simulink model "ManobraOrbital"  (R2023b)
settings: Solver=FixedStepAuto  StartTime=0.0  StopTime=tf  FixedStep=step_modelo  RelTol=1e-3
values from neighbouring files (symbols this model uses):
  mi = 3.9860044189*10^14    (= 398600441890000)    [constantes.m]
undefined symbols (not defined in the file or in its folder): e0_ini, pcoRad, step_modelo, t_man, x0_dot, x0_dot_ini, x0_ini, y0_dot_ini, y0_ini, z0_dot_ini, z0_ini
libraries: simulink x5
settings Model: Creator=rodri  LastModifiedBy=rodri
settings DataIOCC: SaveOutput=off  SaveTime=off
settings ModelReferenceCC: EnableRefExpFcnMdlSchedulingChecks=on

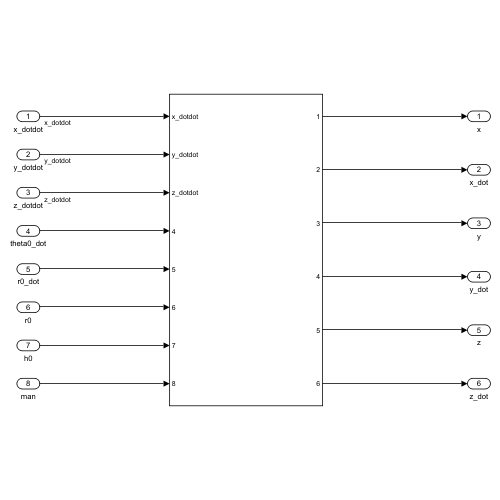
[thumbnail: Simulink's stored preview of the top-level diagram]
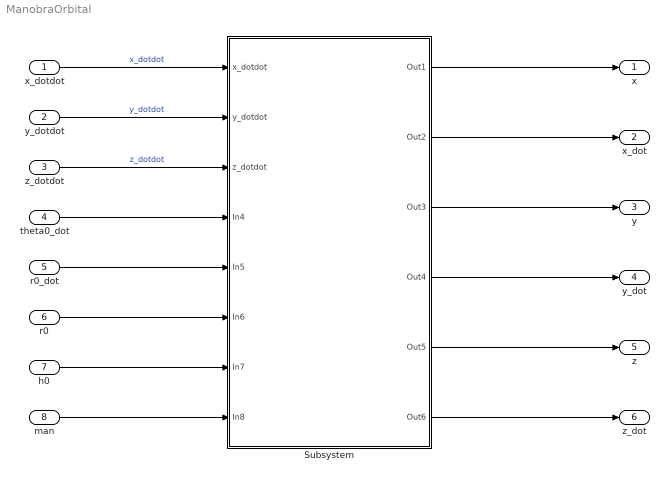
== system ManobraOrbital ==
  x_dotdot : Inport  OutDataTypeStr=double  Interpolate=off
  y_dotdot : Inport  Port=2  OutDataTypeStr=double  Interpolate=off
  z_dotdot : Inport  Port=3  OutDataTypeStr=double  Interpolate=off
  theta0_dot : Inport  Port=4  OutDataTypeStr=double  Interpolate=off
  r0_dot : Inport  Port=5  OutDataTypeStr=double  Interpolate=off
  r0 : Inport  Port=6  OutDataTypeStr=double  Interpolate=off
  h0 : Inport  Port=7  OutDataTypeStr=double  Interpolate=off
  man : Inport  Port=8  OutDataTypeStr=boolean
  Subsystem : Subsystem
  x : Outport  OutDataTypeStr=double
  x_dot : Outport  Port=2  OutDataTypeStr=double
  y : Outport  Port=3  OutDataTypeStr=double
  y_dot : Outport  Port=4  OutDataTypeStr=double
  z : Outport  Port=5  OutDataTypeStr=double
  z_dot : Outport  Port=6  OutDataTypeStr=double
  wires:
  x_dotdot/1 -> Subsystem/1(x_dotdot)  "x_dotdot"
  y_dotdot/1 -> Subsystem/2(y_dotdot)  "y_dotdot"
  z_dotdot/1 -> Subsystem/3(z_dotdot)  "z_dotdot"
  theta0_dot/1 -> Subsystem/4(In4)
  r0_dot/1 -> Subsystem/5(In5)
  r0/1 -> Subsystem/6(In6)
  h0/1 -> Subsystem/7(In7)
  man/1 -> Subsystem/8(In8)
  Subsystem/1(Out1) -> x/1
  Subsystem/2(Out2) -> x_dot/1
  Subsystem/3(Out3) -> y/1
  Subsystem/4(Out4) -> y_dot/1
  Subsystem/5(Out5) -> z/1
  Subsystem/6(Out6) -> z_dot/1

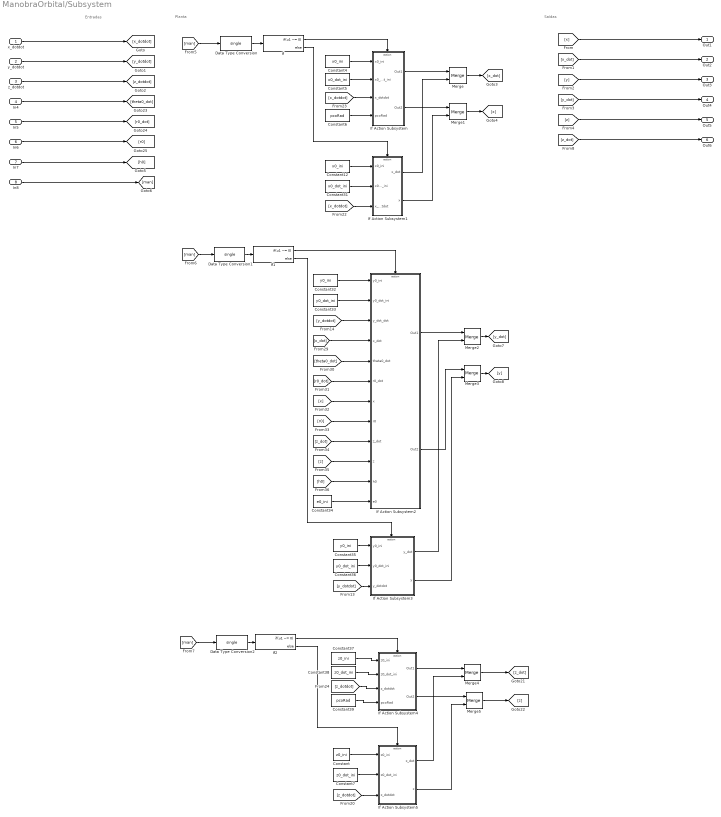
== system ManobraOrbital/Subsystem ==
  note: Planta
  note: Entradas
  note: Saídas
  x_dotdot : Inport
  y_dotdot : Inport  Port=2
  z_dotdot : Inport  Port=3
  In4 : Inport  Port=4
  In5 : Inport  Port=5
  In6 : Inport  Port=6
  In7 : Inport  Port=7
  In8 : Inport  Port=8
  Constant : Constant  Value=z0_ini  SampleTime=-1
  Constant12 : Constant  Value=x0_ini  SampleTime=-1
  Constant31 : Constant  Value=x0_dot_ini  SampleTime=-1
  Constant32 : Constant  Value=y0_ini  SampleTime=-1
  Constant33 : Constant  Value=y0_dot_ini  SampleTime=-1
  Constant34 : Constant  Value=e0_ini  SampleTime=-1  LockScale=on
  Constant35 : Constant  Value=y0_ini  SampleTime=-1
  Constant36 : Constant  Value=y0_dot_ini  SampleTime=-1
  Constant37 : Constant  Value=z0_ini  SampleTime=-1
  Constant38 : Constant  Value=z0_dot_ini  SampleTime=-1
  Constant39 : Constant  Value=pcoRad  SampleTime=-1
  Constant4 : Constant  Value=x0_ini  SampleTime=-1
  Constant5 : Constant  Value=x0_dot_ini  SampleTime=-1
  Constant6 : Constant  Value=pcoRad  SampleTime=-1
  Constant7 : Constant  Value=z0_dot_ini  SampleTime=-1
  Data Type Conversion : DataTypeConversion  OutDataTypeStr=single  SaturateOnIntegerOverflow=off  RndMeth=Floor
  Data Type Conversion1 : DataTypeConversion  OutDataTypeStr=single  SaturateOnIntegerOverflow=off  RndMeth=Floor
  Data Type Conversion2 : DataTypeConversion  OutDataTypeStr=single  SaturateOnIntegerOverflow=off  RndMeth=Floor
  If : If  IfExpression=u1 ~= 0
  If Action Subsystem : Subsystem  TreatAsAtomicUnit=on
  If Action Subsystem1 : Subsystem  TreatAsAtomicUnit=on
  If Action Subsystem2 : Subsystem  TreatAsAtomicUnit=on
  If Action Subsystem3 : Subsystem  TreatAsAtomicUnit=on
  If Action Subsystem4 : Subsystem  TreatAsAtomicUnit=on
  If Action Subsystem5 : Subsystem  TreatAsAtomicUnit=on
  If1 : If  IfExpression=u1 ~= 0
  If2 : If  IfExpression=u1 ~= 0
  Merge : Merge  InitialOutput=x0_dot_ini
  Merge1 : Merge  InitialOutput=x0_ini
  Merge2 : Merge  InitialOutput=y0_dot_ini
  Merge3 : Merge  InitialOutput=y0_ini
  Merge4 : Merge  InitialOutput=z0_dot_ini
  Merge5 : Merge  InitialOutput=z0_ini
  Out1 : Outport
  Out2 : Outport  Port=2
  Out3 : Outport  Port=3
  Out4 : Outport  Port=4
  Out5 : Outport  Port=5
  Out6 : Outport  Port=6
  wires:
  [y_dotdot] -> If Action Subsystem2/3(y_dot_dot)
  Merge/1 -> [x_dot]
  If Action Subsystem4/2(Out2) -> Merge5/1
  Constant5/1 -> If Action Subsystem/2(x0_dot_ini)
  Constant37/1 -> If Action Subsystem4/1(z0_ini)
  [x] -> Out1/1
  Constant7/1 -> If Action Subsystem5/2(z0_dot_ini)
  [r0] -> If Action Subsystem2/8(r0)
  If2/2 -> If Action Subsystem5/Action
  If Action Subsystem/2(Out2) -> Merge1/1
  [z_dotdot] -> If Action Subsystem5/3(z_dotdot)
  [z_dot] -> Out6/1
  Constant32/1 -> If Action Subsystem2/1(y0_ini)
  [h0] -> If Action Subsystem2/11(h0)
  In8/1 -> [man]
  If1/2 -> If Action Subsystem3/Action
  Constant35/1 -> If Action Subsystem3/1(y0_ini)
  If1/1 -> If Action Subsystem2/Action
  [y_dotdot] -> If Action Subsystem3/3(y_dotdot)
  Data Type Conversion2/1 -> If2/1
  If Action Subsystem3/1(y_dot) -> Merge2/2
  In7/1 -> [h0]
  In5/1 -> [r0_dot]
  Merge2/1 -> [y_dot]
  Constant/1 -> If Action Subsystem5/1(z0_ini)
  If2/1 -> If Action Subsystem4/Action
  [r0_dot] -> If Action Subsystem2/6(r0_dot)
  If Action Subsystem1/1(x_dot) -> Merge/2
  [z] -> If Action Subsystem2/10(z)
  Constant34/1 -> If Action Subsystem2/12(e0)
  [x_dot] -> If Action Subsystem2/4(x_dot)
  Constant36/1 -> If Action Subsystem3/2(y0_dot_ini)
  [theta0_dot] -> If Action Subsystem2/5(theta0_dot)
  Data Type Conversion1/1 -> If1/1
  Merge3/1 -> [y]
  [man] -> Data Type Conversion1/1
  Merge1/1 -> [x]
  If Action Subsystem2/1(Out1) -> Merge2/1
  If Action Subsystem4/1(Out1) -> Merge4/1
  Constant38/1 -> If Action Subsystem4/2(z0_dot_ini)
  Merge4/1 -> [z_dot]
  [x_dotdot] -> If Action Subsystem1/3(x_dotdot)
  If Action Subsystem/1(Out1) -> Merge/1
  [z_dotdot] -> If Action Subsystem4/3(z_dotdot)
  [z_dot] -> If Action Subsystem2/9(z_dot)
  If Action Subsystem2/2(Out2) -> Merge3/1
  If Action Subsystem1/2(x) -> Merge1/2
  Constant39/1 -> If Action Subsystem4/4(pcoRad)
  If Action Subsystem3/2(y) -> Merge3/2
  Constant31/1 -> If Action Subsystem1/2(x0_dot_ini)
  Constant4/1 -> If Action Subsystem/1(x0_ini)
  If/1 -> If Action Subsystem/Action
  [man] -> Data Type Conversion/1
  Data Type Conversion/1 -> If/1
  Constant12/1 -> If Action Subsystem1/1(x0_ini)
  Merge5/1 -> [z]
  Constant6/1 -> If Action Subsystem/4(pcoRad)
  If/2 -> If Action Subsystem1/Action
  [x_dot] -> Out2/1
  [x] -> If Action Subsystem2/7(x)
  Constant33/1 -> If Action Subsystem2/2(y0_dot_ini)
  [man] -> Data Type Conversion2/1
  If Action Subsystem5/1(z_dot) -> Merge4/2
  y_dotdot/1 -> [y_dotdot]
  If Action Subsystem5/2(z) -> Merge5/2
  [x_dotdot] -> If Action Subsystem/3(x_dotdot)
  In6/1 -> [r0]
  [z] -> Out5/1
  x_dotdot/1 -> [x_dotdot]
  z_dotdot/1 -> [z_dotdot]
  [y] -> Out3/1
  In4/1 -> [theta0_dot]
  [y_dot] -> Out4/1

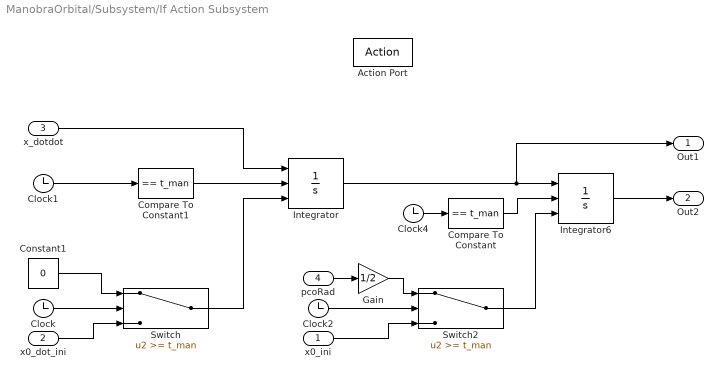
== system ManobraOrbital/Subsystem/If Action Subsystem ==
  x0_ini : Inport
  x0_dot_ini : Inport  Port=2
  x_dotdot : Inport  Port=3
  pcoRad : Inport  Port=4
  Action Port : ActionPort  ActionPortLabel=if(u1 ~= 0)
  Clock{,1..2,4} (4 alike) : Clock
  Compare To Constant : simulink/Logic and Bit Operations/Compare To Constant  relop===  const=t_man  OutDataTypeStr=boolean
  Compare To Constant1 : simulink/Logic and Bit Operations/Compare To Constant  relop===  const=t_man  OutDataTypeStr=boolean
  Constant1 : Constant  Value=0  SampleTime=-1
  Gain : Gain  Gain=1/2
  Integrator : Integrator  ExternalReset=either  InitialConditionSource=external  InitialCondition=x0_dot  AbsoluteTolerance=abs_tol
  Integrator6 : Integrator  ExternalReset=either  InitialConditionSource=external  InitialCondition=x0_dot  AbsoluteTolerance=abs_tol
  Switch : Switch  Threshold=t_man  SaturateOnIntegerOverflow=off  InputSameDT=off
  Switch2 : Switch  Threshold=t_man  SaturateOnIntegerOverflow=off  InputSameDT=off
  Out1 : Outport  InitialOutput=x0_dot_ini
  Out2 : Outport  Port=2  InitialOutput=x0_ini
  wires:
  Integrator6/1 -> Out2/1
  Switch/1 -> Integrator/3
  x_dotdot/1 -> Integrator/1
  Clock/1 -> Switch/2
  Integrator/1 -> Out1/1, Integrator6/1
  Switch2/1 -> Integrator6/3
  x0_dot_ini/1 -> Switch/3
  Compare To Constant/1 -> Integrator6/2
  Compare To Constant1/1 -> Integrator/2
  Constant1/1 -> Switch/1
  Clock2/1 -> Switch2/2
  x0_ini/1 -> Switch2/3
  Clock4/1 -> Compare To Constant/1
  Clock1/1 -> Compare To Constant1/1
  pcoRad/1 -> Gain/1
  Gain/1 -> Switch2/1

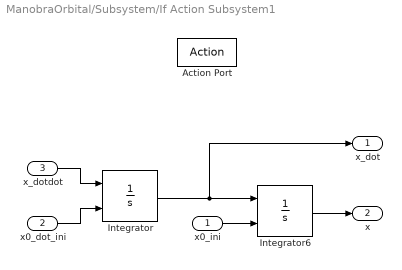
== system ManobraOrbital/Subsystem/If Action Subsystem1 ==
  x0_ini : Inport
  x0_dot_ini : Inport  Port=2
  x_dotdot : Inport  Port=3
  Action Port : ActionPort  ActionPortLabel=else
  Integrator : Integrator  InitialConditionSource=external  InitialCondition=x0_dot  AbsoluteTolerance=abs_tol
  Integrator6 : Integrator  InitialConditionSource=external  InitialCondition=x0_dot  AbsoluteTolerance=abs_tol
  x_dot : Outport  InitialOutput=x0_dot_ini
  x : Outport  Port=2  InitialOutput=x0_ini
  wires:
  x0_ini/1 -> Integrator6/2
  Integrator6/1 -> x/1
  x0_dot_ini/1 -> Integrator/2
  Integrator/1 -> Integrator6/1, x_dot/1
  x_dotdot/1 -> Integrator/1

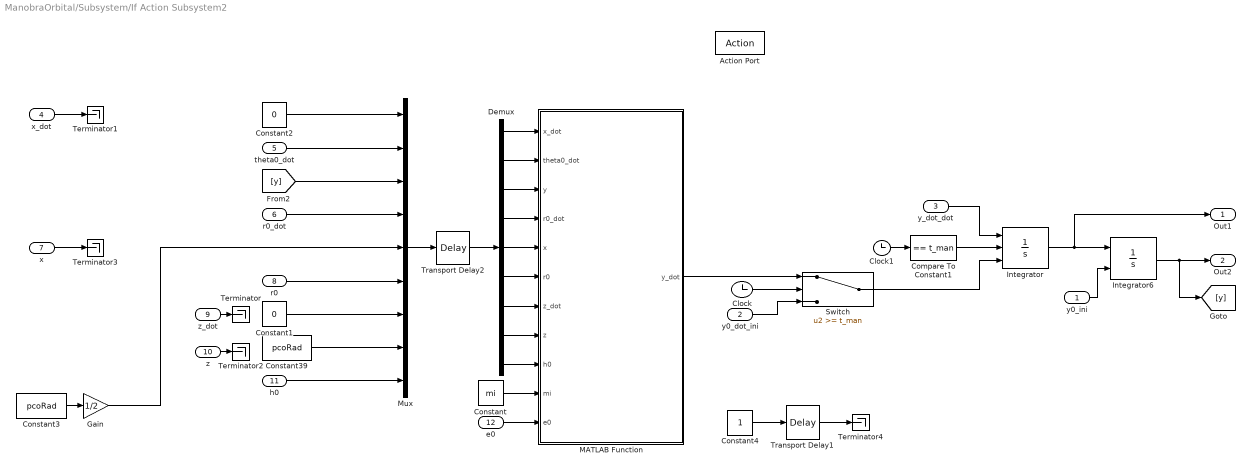
== system ManobraOrbital/Subsystem/If Action Subsystem2 ==
  y0_ini : Inport
  y0_dot_ini : Inport  Port=2
  y_dot_dot : Inport  Port=3
  x_dot : Inport  Port=4
  theta0_dot : Inport  Port=5
  r0_dot : Inport  Port=6
  x : Inport  Port=7
  r0 : Inport  Port=8
  z_dot : Inport  Port=9
  z : Inport  Port=10
  h0 : Inport  Port=11
  e0 : Inport  Port=12
  Action Port : ActionPort  ActionPortLabel=if(u1 ~= 0)
  Clock : Clock
  Clock1 : Clock
  Compare To Constant1 : simulink/Logic and Bit Operations/Compare To Constant  relop===  const=t_man  OutDataTypeStr=boolean
  Constant : Constant  Value=mi  SampleTime=-1
  Constant1 : Constant  Value=0  SampleTime=-1
  Constant2 : Constant  Value=0  SampleTime=-1
  Constant3 : Constant  Value=pcoRad  SampleTime=-1
  Constant39 : Constant  Value=pcoRad  SampleTime=-1
  Constant4 : Constant
  Demux : Demux  Outputs=9
  Gain : Gain  Gain=1/2
  Integrator : Integrator  ExternalReset=either  InitialConditionSource=external  InitialCondition=x0_dot  AbsoluteTolerance=abs_tol
  Integrator6 : Integrator  InitialConditionSource=external  InitialCondition=x0_dot  AbsoluteTolerance=abs_tol
  MATLAB Function : MATLAB Function  TreatAsAtomicUnit=on
  Mux : Mux  Inputs=9
  Switch : Switch  Threshold=t_man  SaturateOnIntegerOverflow=off  InputSameDT=off
  Terminator{,1..4} (5 alike) : Terminator
  Transport Delay1 : TransportDelay  DelayTime=step_modelo
  Transport Delay2 : TransportDelay  DelayTime=step_modelo
  Out1 : Outport  InitialOutput=y0_dot_ini
  Out2 : Outport  Port=2  InitialOutput=y0_ini
  wires:
  Switch/1 -> Integrator/3
  y_dot_dot/1 -> Integrator/1
  Clock/1 -> Switch/2
  Integrator/1 -> Integrator6/1, Out1/1
  y0_ini/1 -> Integrator6/2
  y0_dot_ini/1 -> Switch/3
  Compare To Constant1/1 -> Integrator/2
  MATLAB Function/1(y_dot) -> Switch/1
  Clock1/1 -> Compare To Constant1/1
  Constant/1 -> MATLAB Function/10(mi)
  e0/1 -> MATLAB Function/11(e0)
  Integrator6/1 -> [y], Out2/1
  theta0_dot/1 -> Mux/2
  [y] -> Mux/3
  r0_dot/1 -> Mux/4
  r0/1 -> Mux/6
  h0/1 -> Mux/9
  Demux/9 -> MATLAB Function/9(h0)
  Demux/8 -> MATLAB Function/8(z)
  Demux/7 -> MATLAB Function/7(z_dot)
  Demux/6 -> MATLAB Function/6(r0)
  Demux/5 -> MATLAB Function/5(x)
  Demux/4 -> MATLAB Function/4(r0_dot)
  Demux/3 -> MATLAB Function/3(y)
  Demux/2 -> MATLAB Function/2(theta0_dot)
  Demux/1 -> MATLAB Function/1(x_dot)
  Mux/1 -> Transport Delay2/1
  Constant1/1 -> Mux/7
  z_dot/1 -> Terminator/1
  Constant2/1 -> Mux/1
  x_dot/1 -> Terminator1/1
  Constant39/1 -> Mux/8
  z/1 -> Terminator2/1
  Constant3/1 -> Gain/1
  Gain/1 -> Mux/5
  x/1 -> Terminator3/1
  Constant4/1 -> Transport Delay1/1
  Transport Delay1/1 -> Terminator4/1
  Transport Delay2/1 -> Demux/1

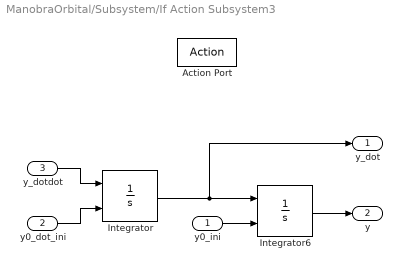
== system ManobraOrbital/Subsystem/If Action Subsystem3 ==
  y0_ini : Inport
  y0_dot_ini : Inport  Port=2
  y_dotdot : Inport  Port=3
  Action Port : ActionPort  ActionPortLabel=else
  Integrator : Integrator  InitialConditionSource=external  InitialCondition=x0_dot  AbsoluteTolerance=abs_tol
  Integrator6 : Integrator  InitialConditionSource=external  InitialCondition=x0_dot  AbsoluteTolerance=abs_tol
  y_dot : Outport  InitialOutput=y0_dot_ini
  y : Outport  Port=2  InitialOutput=y0_ini
  wires:
  y0_ini/1 -> Integrator6/2
  Integrator6/1 -> y/1
  y0_dot_ini/1 -> Integrator/2
  Integrator/1 -> Integrator6/1, y_dot/1
  y_dotdot/1 -> Integrator/1

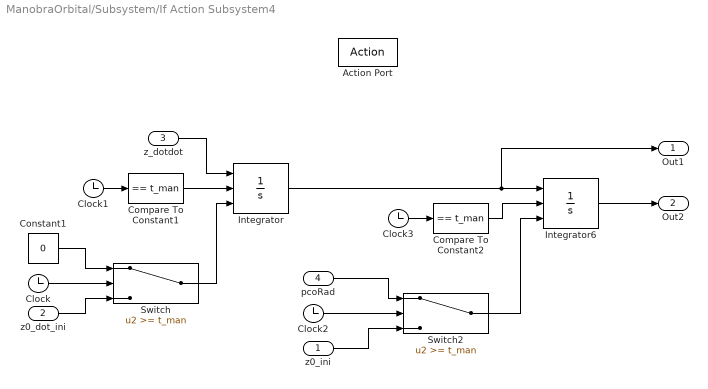
== system ManobraOrbital/Subsystem/If Action Subsystem4 ==
  z0_ini : Inport
  z0_dot_ini : Inport  Port=2
  z_dotdot : Inport  Port=3
  pcoRad : Inport  Port=4
  Action Port : ActionPort  ActionPortLabel=if(u1 ~= 0)
  Clock{,1..3} (4 alike) : Clock
  Compare To Constant1 : simulink/Logic and Bit Operations/Compare To Constant  relop===  const=t_man  OutDataTypeStr=boolean
  Compare To Constant2 : simulink/Logic and Bit Operations/Compare To Constant  relop===  const=t_man  OutDataTypeStr=boolean
  Constant1 : Constant  Value=0  SampleTime=-1
  Integrator : Integrator  ExternalReset=either  InitialConditionSource=external  InitialCondition=x0_dot  AbsoluteTolerance=abs_tol
  Integrator6 : Integrator  ExternalReset=either  InitialConditionSource=external  InitialCondition=x0_dot  AbsoluteTolerance=abs_tol
  Switch : Switch  Threshold=t_man  SaturateOnIntegerOverflow=off  InputSameDT=off
  Switch2 : Switch  Threshold=t_man  SaturateOnIntegerOverflow=off  InputSameDT=off
  Out1 : Outport  InitialOutput=z0_dot_ini
  Out2 : Outport  Port=2  InitialOutput=z0_ini
  wires:
  Integrator6/1 -> Out2/1
  Switch/1 -> Integrator/3
  z_dotdot/1 -> Integrator/1
  Clock/1 -> Switch/2
  Integrator/1 -> Out1/1, Integrator6/1
  Switch2/1 -> Integrator6/3
  z0_dot_ini/1 -> Switch/3
  Compare To Constant2/1 -> Integrator6/2
  Compare To Constant1/1 -> Integrator/2
  pcoRad/1 -> Switch2/1
  Clock2/1 -> Switch2/2
  z0_ini/1 -> Switch2/3
  Clock1/1 -> Compare To Constant1/1
  Clock3/1 -> Compare To Constant2/1
  Constant1/1 -> Switch/1

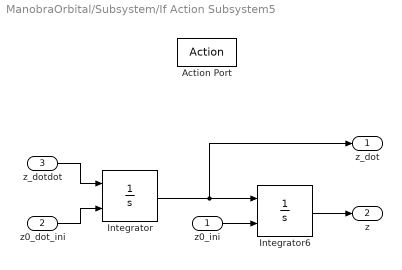
== system ManobraOrbital/Subsystem/If Action Subsystem5 ==
  z0_ini : Inport
  z0_dot_ini : Inport  Port=2
  z_dotdot : Inport  Port=3
  Action Port : ActionPort  ActionPortLabel=else
  Integrator : Integrator  InitialConditionSource=external  InitialCondition=x0_dot  AbsoluteTolerance=abs_tol
  Integrator6 : Integrator  InitialConditionSource=external  InitialCondition=x0_dot  AbsoluteTolerance=abs_tol
  z_dot : Outport  InitialOutput=z0_dot_ini
  z : Outport  Port=2  InitialOutput=z0_ini
  wires:
  z0_ini/1 -> Integrator6/2
  Integrator6/1 -> z/1
  z0_dot_ini/1 -> Integrator/2
  Integrator/1 -> Integrator6/1, z_dot/1
  z_dotdot/1 -> Integrator/1

== matlab function ManobraOrbital/Subsystem/If Action Subsystem2/MATLAB Function ==
  data: x_dot input; y_dot output; theta0_dot input; y input; r0_dot input; x input; r0 input; z_dot input; z input; h0 input; mi input; e0 input
function y_dot = fcn(x_dot,theta0_dot,y,r0_dot,x,r0,z_dot,z,h0,mi,e0)

a0 = (h0^2/mi)/(1 - e0^2);

if ((r0+x)^2+y^2+z^2) < 0
    A1 = 0;
else
    A1 = mi/(sqrt((r0+x)^2+y^2+z^2))-mi/(2*a0);
end

A2 = (x_dot-theta0_dot*y+r0_dot)^2-z_dot^2;

if (2*A1-A2) < 0
    A1 = 0;
    A2 = 0;
end

A3 = theta0_dot*(x+r0);

y_dot = sqrt(2*A1-A2)-A3;
